simulink model "drone_model"  (R2016b)
settings: Solver=VariableStepAuto  StartTime=0.0  StopTime=10.0  RelTol=1e-3
libraries: FMIKit_blocks x1, simulink x1
settings Model: Creator=luigiv  LastModifiedBy=luigiv
settings SFSimCC: SimUserSources="\"\\\\Mac\\Home\\Documents\\MATLAB\\Add-Ons\\Apps\\FMIKit - 2\\code\\src\\FMU.cpp\" \"\\\\Mac\\Home\\Documents\\MATLAB\\Add-Ons\\Apps\\FMIKit - 2\\code\\src\\FMU1.cpp\" \"\\\\Mac\\Home\\Documents\\MATLAB\\Add-Ons\\Apps\\FMIKit - 2\\code\\src\\FMU2.cpp\""  SimUserIncludeDirs="\"\\\\Mac\\Home\\Documents\\MATLAB\\Add-Ons\\Apps\\FMIKit - 2\\code\\include\""  SimUserLibraries="\"C:\\Program Files (x86)\\Microsoft SDKs\\Windows\\v8.1A\\Lib\\x64\\ShLwApi.Lib\""
settings RTWCC: CustomInclude="\"\\\\Mac\\Home\\Documents\\MATLAB\\Add-Ons\\Apps\\FMIKit - 2\\code\\include\""  CustomSource="\"\\\\Mac\\Home\\Documents\\MATLAB\\Add-Ons\\Apps\\FMIKit - 2\\code\\src\\FMU.cpp\" \"\\\\Mac\\Home\\Documents\\MATLAB\\Add-Ons\\Apps\\FMIKit - 2\\code\\src\\FMU1.cpp\" \"\\\\Mac\\Home\\Documents\\MATLAB\\Add-Ons\\Apps\\FMIKit - 2\\code\\src\\FMU2.cpp\""  CustomLibrary="\"C:\\Program Files (x86)\\Microsoft SDKs\\Windows\\v8.1A\\Lib\\x64\\ShLwApi.Lib\""

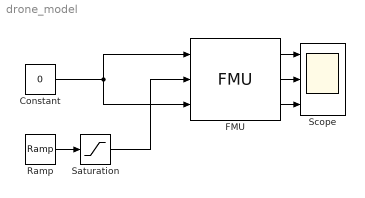
== system drone_model ==
  Constant : Constant  Value=0
  FMU : FMIKit_blocks/FMU
  Ramp : simulink/Sources/Ramp  slope=1  start=0  X0=0
  Saturation : Saturate  UpperLimit=5  LowerLimit=0
  Scope : Scope  NumInputPorts=3
  wires:
  Constant/1 -> FMU/3, FMU/1
  Ramp/1 -> Saturation/1
  Saturation/1 -> FMU/2
  FMU/3 -> Scope/3
  FMU/2 -> Scope/2
  FMU/1 -> Scope/1
